simulink model "MATE_SynchronousMachine"  (R2024b)
settings: Solver=FixedStepDiscrete  StartTime=0.0  StopTime=6  FixedStep=Ts  RelTol=1e-4  EnableMultiTasking=on
PostLoadFcn:
  | Ts=25e-6;offset=4;
InitFcn:
  | Ts=25e-6;offset=4;
undefined symbols (not defined in the file): DiscIntNeverNeededParam, MATE, Phase, Rsnu, Single
libraries: fl_lib x79, nesl_utility x53, ee_lib x16, simetran x5, powerlib_extras x3, simulink_extras x2, simulink x2
(part 3 of 5)

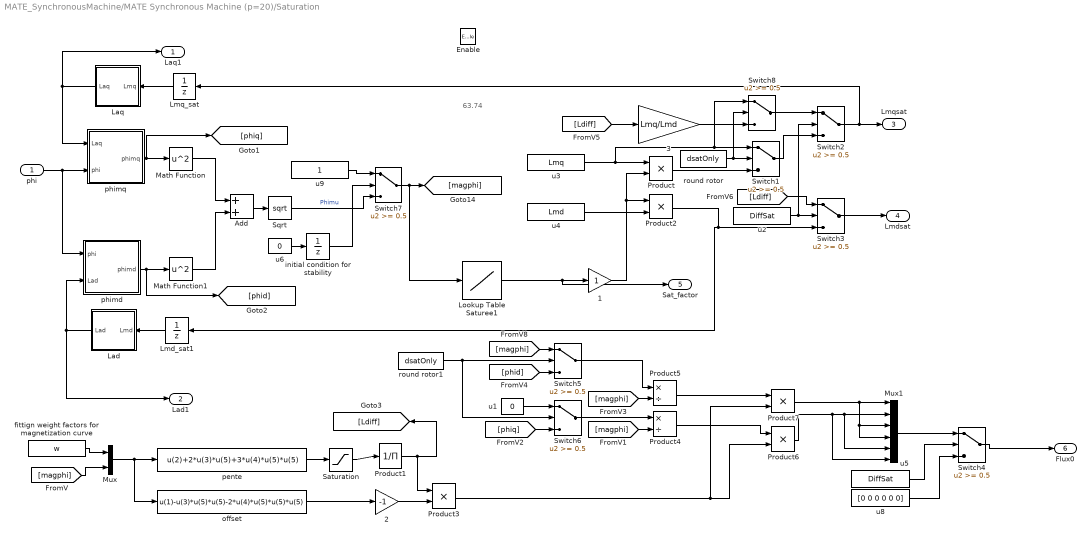
== system MATE_SynchronousMachine/MATE Synchronous Machine (p=20)/Saturation ==
  note: 63.74
  phi : Inport
  Enable : EnablePort
  1 : Gain  SaturateOnIntegerOverflow=on  OutDataTypeStr=Inherit: Same as input  ParamDataTypeStr=Inherit: Same as input
  2 : Gain  Gain=-1  SaturateOnIntegerOverflow=on  OutDataTypeStr=Inherit: Same as input  ParamDataTypeStr=Inherit: Same as input
  3 : Gain  Gain=Lmq/Lmd  SaturateOnIntegerOverflow=on  OutDataTypeStr=Inherit: Same as input  ParamDataTypeStr=Inherit: Same as input
  Add : Sum
  Lad : Subsystem
  Laq : Subsystem
  Lmd_sat1 : UnitDelay  InitialCondition=Lmd  SampleTime=Ts  HasFrameUpgradeWarning=on
  Lmq_sat : UnitDelay  InitialCondition=Lmq  SampleTime=Ts  HasFrameUpgradeWarning=on
  Lookup Table Saturee1 : Lookup  InputValues=table_flux_input  Table=table_saturation_factor  SaturateOnIntegerOverflow=off
  Math Function : Math  Operator=square  SignedPower=on
  Math Function1 : Math  Operator=square  SignedPower=on
  Mux : Mux  Inputs=2
  Mux1 : Mux  Inputs=6
  Product{,2..3,6..7} (5 alike) : Product  RndMeth=Zero
  Product1 : Product  Inputs=/  RndMeth=Zero
  Product4 : Product  Inputs=*/  RndMeth=Zero
  Product5 : Product  Inputs=*/  RndMeth=Zero
  Saturation : Saturate  UpperLimit=inf  LowerLimit=1e-7
  Sqrt : Sqrt  OutputSignalType=real
  Switch{1..8} (8 alike) : Switch  Threshold=0.5  SaturateOnIntegerOverflow=off  InputSameDT=off
  fittign weight factors for magnetization curve : Constant  Value=w
  initial condition for stability : UnitDelay  InitialCondition=1  SampleTime=Ts  HasFrameUpgradeWarning=on
  offset : Fcn  Expr=u(1)-u(3)*u(5)*u(5)-2*u(4)*u(5)*u(5)*u(5)
  pente : Fcn  Expr=u(2)+2*u(3)*u(5)+3*u(4)*u(5)*u(5)
  phimd : Subsystem
  phimq : Subsystem
  round rotor : Constant  Value=dsatOnly
  round rotor1 : Constant  Value=dsatOnly
  u1 : Constant  Value=0
  u2 : Constant  Value=DiffSat
  u3 : Constant  Value=Lmq
  u4 : Constant  Value=Lmd
  u5 : Constant  Value=DiffSat
  u6 : Constant  Value=0
  u8 : Constant  Value=[0 0 0 0 0 0]
  u9 : Constant
  Laq1 : Outport
  Lad1 : Outport  Port=2
  Lmqsat : Outport  Port=3
  Lmdsat : Outport  Port=4
  Sat_factor : Outport  Port=5
  Flux0 : Outport  Port=6
  wires:
  u6/1 -> initial condition for stability/1
  Product2/1 -> Lmd_sat1/1, Switch3/3
  u4/1 -> Product2/2
  u3/1 -> Product/1, Switch1/1, Switch8/1
  Sqrt/1 -> Switch7/3  "Phimu"
  Math Function1/1 -> Add/2
  Math Function/1 -> Add/1
  Add/1 -> Sqrt/1
  phi/1 -> phimd/1(phi), phimq/2(phi)
  Lad/1(Lad) -> Lad1/1, phimd/2(Lad)
  phimd/1(phimd) -> [phid], Math Function1/1
  Lmd_sat1/1 -> Lad/1(Lmd)
  Laq/1(Laq) -> phimq/1(Laq), Laq1/1
  phimq/1(phimq) -> [phiq], Math Function/1
  Lmq_sat/1 -> Laq/1(Lmq)
  round rotor/1 -> Switch1/2, Switch8/2
  Product/1 -> Switch1/3
  Switch1/1 -> Switch2/3
  1/1 -> Product/2, Product2/1
  Lookup Table Saturee1/1 -> 1/1, Sat_factor/1
  fittign weight factors for magnetization curve/1 -> Mux/1
  [magphi] -> Mux/2
  Mux/1 -> pente/1, offset/1
  Product1/1 -> [Ldiff], Product3/1
  offset/1 -> 2/1
  2/1 -> Product3/2
  Product3/1 -> Product7/2, Product6/2
  [magphi] -> Product4/2
  [magphi] -> Product5/2
  Product6/1 -> Mux1/2, Mux1/5, Mux1/6
  Product7/1 -> Mux1/1, Mux1/3, Mux1/4
  Product5/1 -> Product7/1
  Product4/1 -> Product6/1
  Switch3/1 -> Lmdsat/1
  Switch2/1 -> Lmq_sat/1, Lmqsat/1
  u2/1 -> Switch3/2, Switch2/2
  [Ldiff] -> 3/1
  [Ldiff] -> Switch3/1
  Mux1/1 -> Switch4/1
  Switch4/1 -> Flux0/1
  u5/1 -> Switch4/2
  u8/1 -> Switch4/3
  pente/1 -> Saturation/1
  Saturation/1 -> Product1/1
  u9/1 -> Switch7/1
  Switch7/1 -> [magphi], Lookup Table Saturee1/1
  initial condition for stability/1 -> Switch7/2
  [phid] -> Switch5/3
  [phiq] -> Switch6/3
  Switch5/1 -> Product5/1
  Switch6/1 -> Product4/1
  [magphi] -> Switch5/1
  u1/1 -> Switch6/1
  round rotor1/1 -> Switch6/2, Switch5/2
  Switch8/1 -> Switch2/1
  3/1 -> Switch8/3

== system MATE_SynchronousMachine/MATE Synchronous Machine (p=20)/Update Matrix L (with Lcanay) ==
  Lmq : Inport
  Lmd : Inport  Port=2
  Ll : Inport  Port=3
  Selector1 : Selector  NumberOfDimensions=2  InputPortWidth=3  IndexOptions=Index vector (dialog),Index vector (dialog)  Indices=[1:nb_row],[1:nb_row]  OutputSizes=1,1
  Selector8 : Selector  NumberOfDimensions=2  InputPortWidth=3  IndexOptions=Index vector (dialog),Index vector (dialog)  Indices=[1:nb_row],[1:nb_row]  OutputSizes=1,1
  Sum1 : Sum  SaturateOnIntegerOverflow=on
  Sum2 : Sum  SaturateOnIntegerOverflow=on
  Update Lmd rows[1] col[1] : Assignment  NumberOfDimensions=2  IndexOptions=Index vector (dialog),Index vector (dialog)  Indices=[1 3 4],[1 3 4]  OutputSizes=1,1
  "Update Lmq rows[1,5, (6)] col[1,5, (6)] " : Assignment  NumberOfDimensions=2  IndexOptions=Index vector (dialog),Index vector (dialog)  Indices=[2 5 6],[2 5 6]  OutputSizes=1,1
  u1 : Constant  Value="[0 0 0 0 0 0; 0 0 0 0 0 0; 0 0 Lcanay Lcanay 0 0; 0 0 Lcanay Lcanay 0 0; 0 0 0 0 0 0; 0 0  0 0 0 0]"
  u3 : Constant  Value=zeros(6,6)
  Lsat : Outport
  wires:
  Sum1/1 -> Sum2/1
  Update Lmd rows[1] col[1]/1 -> Sum1/1
  Selector1/1 -> Sum1/2
  u1/1 -> Selector1/1
  "Update Lmq rows[1,5, (6)] col[1,5, (6)] "/1 -> Selector8/1
  Lmq/1 -> "Update Lmq rows[1,5, (6)] col[1,5, (6)] "/2
  u3/1 -> "Update Lmq rows[1,5, (6)] col[1,5, (6)] "/1
  Lmd/1 -> Update Lmd rows[1] col[1]/2
  Ll/1 -> Sum2/2
  Sum2/1 -> Lsat/1
  Selector8/1 -> Update Lmd rows[1] col[1]/1

== system MATE_SynchronousMachine/MATE Synchronous Machine (p=20)/inverse ==
  Lsat : Inport
  Enable : EnablePort
  Gain8 : Gain  Gain=-1
  Goto1 : Goto  Commented=on  GotoTag=invL
  Product3 : Product  Multiplication=Matrix(*)  SaturateOnIntegerOverflow=on  OutDataTypeStr=Inherit: Same as first input
  Rwinding : Constant  Value="[Rs 0 0 0 0 0; 0 Rs 0 0 0 0; 0 0 Rf  0 0 0; 0 0 0 Rkd 0 0; 0 0 0 0  Rkq 0; 0 0 0 0 0 Rkq2]"
  Selector8 : Selector  NumberOfDimensions=2  InputPortWidth=3  IndexOptions=Index vector (dialog),Index vector (dialog)  Indices=[1:nb_row],[1:nb_row]  OutputSizes=1,1
  inversion2 : Product  Inputs=/  Multiplication=Matrix(*)  RndMeth=Zero
  -R*inv(L) : Outport
  inv(L) : Outport  Port=2
  wires:
  Gain8/1 -> Product3/1
  inversion2/1 -> Goto1/1, Product3/2, inv(L)/1
  Lsat/1 -> inversion2/1
  Selector8/1 -> Gain8/1
  Rwinding/1 -> Selector8/1
  Product3/1 -> -R*inv(L)/1

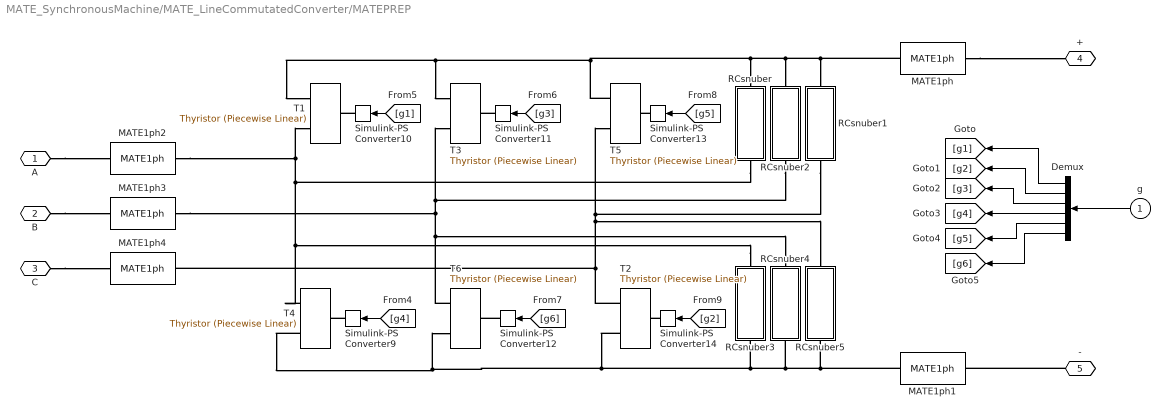
== system MATE_SynchronousMachine/MATE_LineCommutatedConverter/MATEPREP ==
  g : Inport
  Demux : Demux  Outputs=6
  MATE1ph : simetran/MATE1ph  bn=4  conty=Single-Phase  it=auto  Rse=1e-4  Rsh=1e9
      settings: AttributesFormatString=# %<bn>
  MATE1ph1 : simetran/MATE1ph  bn=5  conty=Single-Phase  it=auto  Rse=1e-4  Rsh=1e9
      settings: AttributesFormatString=# %<bn>
  MATE1ph2 : simetran/MATE1ph  bn=1  conty=Single-Phase  it=auto  Rse=1e-4  Rsh=1e9
      settings: AttributesFormatString=# %<bn>
  MATE1ph3 : simetran/MATE1ph  bn=2  conty=Single-Phase  it=auto  Rse=1e-4  Rsh=1e9
      settings: AttributesFormatString=# %<bn>
  MATE1ph4 : simetran/MATE1ph  bn=3  conty=Single-Phase  it=auto  Rse=1e-4  Rsh=1e9
      settings: AttributesFormatString=# %<bn>
  RCsnuber : Subsystem
  RCsnuber1 : Subsystem
  RCsnuber2 : Subsystem
  RCsnuber3 : Subsystem
  RCsnuber4 : Subsystem
  RCsnuber5 : Subsystem
  Simulink-PS Converter{9..14} (6 alike) : nesl_utility/Simulink-PS Converter  PhysicalDomain=network_engine_domain  SubClassName=ps_input  LeftPortType=input  RightPortType=output  PseudoPeriodic=off  Frequencies=[]  NoiseDistribution=none  NoiseParameters=[]  Unit=1  AffineConversion=off  FilteringAndDerivatives=provide  SimscapeFilterOrder=1  InputFilterTimeConstant=0.001  UdotUserProvided=0
  T{1..6} (6 alike) : ee_lib/Semiconductors & Converters/Thyristor (Piecewise Linear)  port_option=ee.enum.controlport.ps  Vf=0.8 V  Ron=0.001 Ohm  Goff=1e-5 1/Ohm  Vgt=0.5 V  Ih=1 A  diode_param=ee.enum.semiconductors.protectionDiode.external  diode_Vf=0.8 V  diode_Ron=0.001 Ohm  diode_Goff=1e-5 1/Ohm  diode_C=50e-9 F  diode_iRM=-235 A  diode_iF=300 A  diode_idot=-50 A/us  diode_trr_param=ee.enum.converters.diodetrr.trr_factor  diode_trr_factor=3  diode_trr=15 us  diode_Qrr=1500 s*uA  iak_specify=off  iak_priority=None  iak=0 A  iak_nominal_specify=off  iak_nominal_value=1  iak_nominal_unit=A  vak_specify=off  vak_priority=None  vak=0 V  vak_nominal_specify=off  vak_nominal_value=1  vak_nominal_unit=V  vgk_specify=off  vgk_priority=None  vgk=0 V  vgk_nominal_specify=off  vgk_nominal_value=1  vgk_nominal_unit=V  thermal_loss_option=ee.enum.converters.thermalLossOption.constantvalues  Von_data=[0, .1, .6, .8, 1, 1.3, 1.6, 2, 2.4; 0, .1, .7, 1, 1.2, 1.5, 1.9, 2.4, 2.8] V  Tj=[298.15, 398.15] K  Iout_data=[0, .1, 1, 5, 10, 20, 40, 70, 100] A  Eon_data=[0, .0024, .024, .12, .2, .48, 1.04, 2.16, 3.24; 0, .003, .03, .15, .25, .6, 1.3, 2.7, 4.05] * 1e-3 J  Tj_loss=[298.15, 398.15] K  Iout_data_loss=[0, .1, 1, 5, 10, 20, 40, 70, 100] A  Eon_scalar=22.86e-3 J  Eoff_natural_commutation=10e-3 J  Voff=300 V  Iout_scalar=600 A  onCurrentMeasDelay=1e-4 s  diodeModelType=ee.enum.converters.diodeModelType.pwl  diodeTableType=ee.enum.diode.tableType.IfMat  diode_IfMat=[.07, .12, .19, 1.75, 4.24, 7.32, 11.2; .16, .3, .72, 2.14, 4.02, 6.35, 9.12] A  diode_VfMat=[.9, 1.15, 1.25, 1.5, 1.75, 2.17, 2.6, 2.85; .58, .68, .75, 1.1, 1.38, 1.77, 2.27, 2.7] V  diode_TjVec=[25, 125] degC  diode_VfVec=[.5, .7, .9, 1.3, 1.7, 2.1, 2.5] V  diode_IfVec=[.1, .2, .5, 1, 2, 4, 7, 10] A  diode_rec_loss_model=ee.enum.diode.reverseRecoveryModel.fixed  diode_ErecVal=0 J  diode_scaleWithIandV=true  diode_ErecMat=zeros(2, 3) J  diode_TjrecVec=[298.15, 398.15] K  diode_IfrecVec=[.1, 1, 10] A  diode_IrecVal=10 A  diode_VrecVal=10 V  diode_tFilter=1 / 1000 / 100 s  thermal_network_parameterization=ee.enum.thermalNetworkTopology.external  Rth=[.08, .5] K/W  Rth_Cauer=[.08, .1, .5] K/W  Rth_Foster=[.08, .14, .22, .16] K/W  thermal_mass_parameterization=ee.enum.thermalNetwork.timeconstant  thermal_mass=[.01, .5] J/K  thermal_mass_Cauer=[.01, .1, .5] J/K  thermal_mass_Foster=[.001, .005, .05, .5] J/K  thermal_time_constant=[.001, .2] s  thermal_time_constant_Cauer=[.001, .1, .2] s  thermal_time_constant_Foster=[7e-05, .0007, .01, .08] s  thermal_mass_initial_temperatures=[25, 25] degC  thermal_mass_initial_temperatures_Cauer=[25, 25, 25] degC  junction_thermal_mass=0.01 J/K  Tvec_initial_Foster=[25, 25, 25, 25] degC  junction_temperature_specify=off  junction_temperature_priority=None  junction_temperature=25 degC  junction_temperature_nominal_specify=off  junction_temperature_nominal_value=1  junction_temperature_nominal_unit=degC  Qj_specify=off  Qj_priority=None  Qj=0 W  Qj_nominal_specify=off  Qj_nominal_value=1  Qj_nominal_unit=W  accumulatedSwitchingLosses_specify=off  accumulatedSwitchingLosses_priority=None  accumulatedSwitchingLosses=0 J
      settings: InternalSimscapePortConfiguration="{\"Bottom\":[],\"Left\":[{\"id\":\"G\",\"label\":\"\",\"type\":\"input\"}],\"Right\":[{\"id\":\"A\",\"label\":\"\",\"type\":\"foundation.electrical.electrical\"},{\"id\":\"K\",\"label\":\"\",\"type\":\"foundation.electrical.electrical\"}],\"Top\":[]}"
  A : PMIOPort  Side=Left
  B : PMIOPort  Port=2  Side=Left
  C : PMIOPort  Port=3  Side=Left
  + : PMIOPort  Port=4  Side=Right
  - : PMIOPort  Port=5  Side=Right
  wires:
  Demux/5 -> [g5]
  Demux/6 -> [g6]
  Demux/4 -> [g4]
  Demux/3 -> [g3]
  Demux/2 -> [g2]
  Demux/1 -> [g1]
  g/1 -> Demux/1
  [g4] -> Simulink-PS Converter9/1
  [g1] -> Simulink-PS Converter10/1
  [g3] -> Simulink-PS Converter11/1
  [g6] -> Simulink-PS Converter12/1
  [g5] -> Simulink-PS Converter13/1
  [g2] -> Simulink-PS Converter14/1
  connections:
  RCsnuber3/LConn1 -- T4/RConn2 -- RCsnuber/RConn1 -- MATE1ph2/RConn1 -- T1/RConn1
  MATE1ph3/RConn1 -- RCsnuber2/RConn1 -- T3/RConn1 -- T6/RConn2 -- RCsnuber4/LConn1
  RCsnuber1/RConn1 -- T5/RConn1 -- T2/RConn2 -- MATE1ph4/RConn1 -- RCsnuber5/LConn1
  RCsnuber4/RConn1 -- MATE1ph1/RConn1 -- RCsnuber5/RConn1 -- T2/RConn1 -- T6/RConn1 -- T4/RConn1 -- RCsnuber3/RConn1
  MATE1ph/RConn1 -- T1/RConn2 -- T3/RConn2 -- T5/RConn2 -- RCsnuber/LConn1 -- RCsnuber2/LConn1 -- RCsnuber1/LConn1
  -/RConn1 -- MATE1ph1/LConn1
  A/RConn1 -- MATE1ph2/LConn1
  B/RConn1 -- MATE1ph3/LConn1
  C/RConn1 -- MATE1ph4/LConn1
  Simulink-PS Converter9/RConn1 -- T4/LConn1
  Simulink-PS Converter10/RConn1 -- T1/LConn1
  Simulink-PS Converter11/RConn1 -- T3/LConn1
  Simulink-PS Converter12/RConn1 -- T6/LConn1
  Simulink-PS Converter13/RConn1 -- T5/LConn1
  Simulink-PS Converter14/RConn1 -- T2/LConn1
  MATE1ph/LConn1 -- +/RConn1

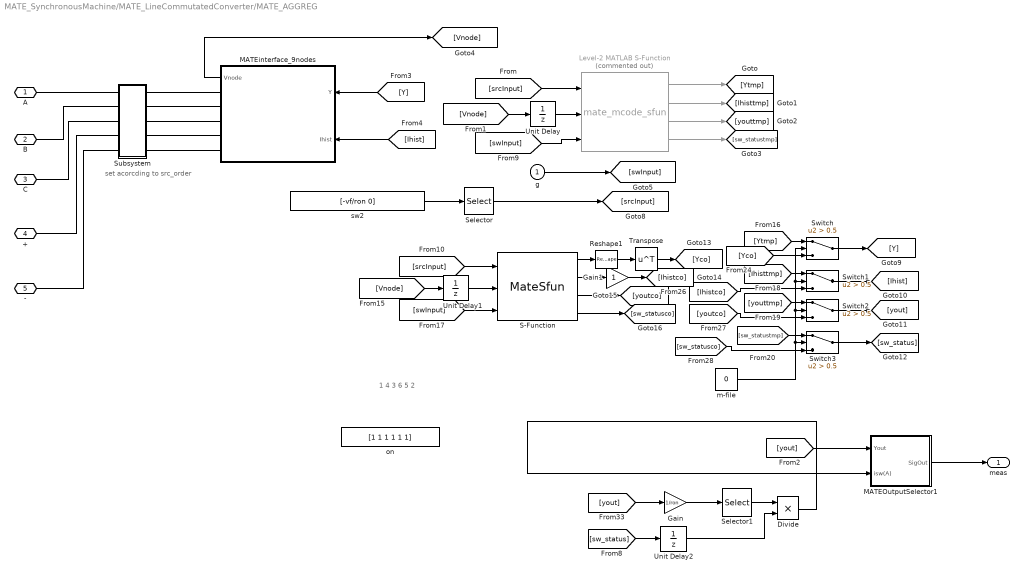
== system MATE_SynchronousMachine/MATE_LineCommutatedConverter/MATE_AGGREG ==
  note: set acorcding to src_order
  note: 1 4 3 6 5 2
  g : Inport
  Divide : Product
  Gain : Gain  Gain=1/ron
  Gain1 : Gain
  Level-2 MATLAB S-Function : M-S-Function  Commented=on  FunctionName=mate_mcode_sfun  Parameters=MATE,vf
  MATEOutputSelector1 : Subsystem
  MATEinterface_9nodes : Subsystem
  Reshape1 : Reshape  OutputDimensionality=Customize  OutputDimensions=[MATE.NumberOfNodes,MATE.NumberOfNodes]
  S-Function : S-Function  FunctionName=MateSfun  Parameters="MATERT.sizes,MATERT.As  ,MATERT.Bs,MATERT.Cs,MATERT.Ds,MATERT.Rsw,MATERT.SwType,MATERT.DISC,MATERT.h,MATERT.U0,MATERT.X0,vf"  SFunctionDeploymentMode=off  EnableBusSupport=off
  Selector : Selector  InputPortWidth=2  IndexOptions=Index vector (dialog)  Indices="[1 1 1 1 1 1  2 2 2 2 2]"  OutputSizes=1
  Selector1 : Selector  InputPortWidth=11  IndexOptions=Index vector (dialog)  Indices=[1 2 3 4 5 6]  OutputSizes=1
  Subsystem : Subsystem
  Switch{,1..3} (4 alike) : Switch  Criteria=u2 > Threshold  Threshold=0.5  SaturateOnIntegerOverflow=off  InputSameDT=off
  Transpose : Math  Operator=transpose
  Unit Delay : UnitDelay  SampleTime=Ts  HasFrameUpgradeWarning=on
  Unit Delay1 : UnitDelay  SampleTime=Ts  HasFrameUpgradeWarning=on
  Unit Delay2 : UnitDelay  SampleTime=Ts  HasFrameUpgradeWarning=on
  m-file : Constant  Value=0
  on : Constant  Value=[1 1 1 1 1 1]
  sw2 : Constant  Value=[-vf/ron 0]
  A : PMIOPort  Side=Left
  B : PMIOPort  Port=2  Side=Left
  C : PMIOPort  Port=3  Side=Left
  + : PMIOPort  Port=4  Side=Right
  - : PMIOPort  Port=5  Side=Right
  meas : Outport
  wires:
  m-file/1 -> Switch3/2, Switch/2, Switch1/2, Switch2/2
  Level-2 MATLAB S-Function/1 -> [Ytmp]
  Unit Delay/1 -> Level-2 MATLAB S-Function/2
  [swInput] -> S-Function/3
  S-Function/3 -> [youtco]
  Level-2 MATLAB S-Function/2 -> [Ihisttmp]
  Level-2 MATLAB S-Function/3 -> [youttmp]
  [youtco] -> Switch2/3
  [sw_statustmp] -> Switch3/1
  [Vnode] -> Unit Delay1/1
  [youttmp] -> Switch2/1
  [srcInput] -> Level-2 MATLAB S-Function/1
  Gain1/1 -> [Ihistco]
  [Ihistco] -> Switch1/3
  [Ytmp] -> Switch/1
  [Ihist] -> MATEinterface_9nodes/2(Ihist)
  [Vnode] -> Unit Delay/1
  [srcInput] -> S-Function/1
  Unit Delay1/1 -> S-Function/2
  S-Function/1 -> Reshape1/1
  S-Function/2 -> Gain1/1
  Switch2/1 -> [yout]
  Transpose/1 -> [Yco]
  Reshape1/1 -> Transpose/1
  S-Function/4 -> [sw_statusco]
  Switch/1 -> [Y]
  [Ihisttmp] -> Switch1/1
  [sw_statusco] -> Switch3/3
  MATEinterface_9nodes/1(Vnode) -> [Vnode]
  [swInput] -> Level-2 MATLAB S-Function/3
  [Yco] -> Switch/3
  Switch1/1 -> [Ihist]
  [Y] -> MATEinterface_9nodes/1(Y)
  Switch3/1 -> [sw_status]
  Level-2 MATLAB S-Function/4 -> [sw_statustmp]
  sw2/1 -> Selector/1
  Selector/1 -> [srcInput]
  Divide/1 -> MATEOutputSelector1/2(isw(A))
  Selector1/1 -> Divide/1
  [sw_status] -> Unit Delay2/1
  [yout] -> MATEOutputSelector1/1(Yout)
  Gain/1 -> Selector1/1
  Unit Delay2/1 -> Divide/2
  [yout] -> Gain/1
  MATEOutputSelector1/1(SigOut) -> meas/1
  g/1 -> [swInput]
  connections:
  Subsystem/RConn1 -- MATEinterface_9nodes/RConn1
  B/RConn1 -- Subsystem/LConn2
  A/RConn1 -- Subsystem/LConn1
  C/RConn1 -- Subsystem/LConn3
  +/RConn1 -- Subsystem/LConn4
  -/RConn1 -- Subsystem/LConn5
  Subsystem/RConn2 -- MATEinterface_9nodes/RConn2
  Subsystem/RConn3 -- MATEinterface_9nodes/RConn3
  Subsystem/RConn4 -- MATEinterface_9nodes/RConn4
  Subsystem/RConn5 -- MATEinterface_9nodes/RConn5

== system MATE_SynchronousMachine/Mesure et visualisation/Discrete Mean value ==
  In : Inport
  Constant : Constant  Value=Vinit  SampleTime=Ts
  Discrete Variable Transport Delay : powerlib_extras/Discrete  Control Blocks/Discrete Variable Transport Delay  MaxDelay=Delay+Ts  InitialValue=0  Ts=Ts
  Gain : Gain  Gain=K1  SaturateOnIntegerOverflow=on  OutDataTypeStr=Inherit: Same as input  ParamDataTypeStr=Inherit: Same as input
  Gain1 : Gain  Gain=K2  SaturateOnIntegerOverflow=on  OutDataTypeStr=Inherit: Same as input  ParamDataTypeStr=Inherit: Same as input
  Integ4 : DiscreteIntegrator  IntegratorMethod=Integration: Trapezoidal  SampleTime=Ts  ICPrevOutput=DiscIntNeverNeededParam  ICPrevScaledInput=DiscIntNeverNeededParam
  K1 : Constant  Value=Delay  SampleTime=Ts
  K2 : Constant  Value=Freq  SampleTime=Ts
  Product : Product  InputSameDT=on  SaturateOnIntegerOverflow=on  OutDataTypeStr=Inherit: Same as first input
  Step : Step  Time=1/Freq  SampleTime=Ts
  Sum1 : Sum  Inputs=+-  InputSameDT=on  SaturateOnIntegerOverflow=on  OutDataTypeStr=Inherit: Same as first input
  Sum5 : Sum  InputSameDT=on  SaturateOnIntegerOverflow=on  OutDataTypeStr=Inherit: Same as first input
  Sum7 : Sum  Inputs=-+  InputSameDT=on  SaturateOnIntegerOverflow=on  OutDataTypeStr=Inherit: Same as first input
  Switch : Switch  Threshold=0.5  SaturateOnIntegerOverflow=off
  Unit Delay : UnitDelay  SampleTime=Ts  HasFrameUpgradeWarning=on
  Mean : Outport  VectorParamsAs1DForOutWhenUnconnected=off
  wires:
  Product/1 -> Sum5/1  "Mean value"
  Sum7/1 -> Product/1
  Integ4/1 -> Discrete Variable Transport Delay/1, Sum7/2
  K2/1 -> Product/2
  In/1 -> Integ4/1, Gain1/1, Unit Delay/1  "In"
  Sum5/1 -> Switch/1
  Step/1 -> Switch/2
  Constant/1 -> Switch/3
  Switch/1 -> Mean/1
  Discrete Variable Transport Delay/1 -> Sum7/1
  K1/1 -> Discrete Variable Transport Delay/2
  Gain1/1 -> Sum1/1
  Unit Delay/1 -> Gain/1
  Gain/1 -> Sum1/2
  Sum1/1 -> Sum5/2  "Correction"

== system MATE_SynchronousMachine/turbine1/Hydraulic Turbine and Governor ==
  wref : Inport
  Pref : Inport  Port=2
  we : Inport  Port=3
  Pe0 : Inport  Port=4
  dw : Inport  Port=5
  Model : Subsystem  mask(Discrete Hydraulic Turbine and Governor){sm=sm, gate=gate, reg=reg, hyd=hyd, dref=dref, po=po, Ts=Ts}
      mask prompts: sm "Servo-motor [ Ka()  Ta(sec) ]:"; gate "Gate opening limits [ gmin,gmax(pu)    vgmin,vgmax(pu/s) ]:"; reg "Permanent droop and regulator  [ Rp() Kp() Ki() Kd() Td(s) ]:"; hyd "Hydraulic turbine [ beta()  Tw(sec) ]:"; dref "Droop reference (0=power error, 1=gate opening):"; po "Initial mechanical power (pu):"; Ts "Sample time:"
      mask help:
      | Implements a discrete hydraulic turbine combined to a discrete PID governor system.
      |
      | 1st input: desired speed (p.u.);
      | 2nd input: desired electrical power (p.u.);
      | 3rd input: synchronous machine's actual speed (p.u., measurement output 13 of SM block);
      | 4th input: synchronous machine's actual electrical power (p.u., measurement output 14 of SM block);
      | 5th input: synchronous machine's actual speed deviation with respect to nominal (%, measurement output 15 of SM block);
      |
      | 1st output: mechanical power to be applied to the Synchronous Machine block's 1st input (p.u.);
      | 2nd output: gate opening (p.u.).
      mask init:
      | ka=sm(1);ta=sm(2);gmin=gate(1);gmax=gate(2);vgmin=gate(3);vgmax=gate(4);Rp=reg(1);kp=reg(2);ki=reg(3);kd=reg(4);td=reg(5);beta=hyd(1);tw=hyd(2);go=po*(gmax-gmin);
      mask Help: helpview(psbhelp);
  Pm : Outport  InitialOutput=0  VectorParamsAs1DForOutWhenUnconnected=off
  gate : Outport  Port=2  InitialOutput=0  VectorParamsAs1DForOutWhenUnconnected=off
  wires:
  wref/1 -> Model/1(wref)
  Pref/1 -> Model/2(Pref)
  we/1 -> Model/3(we)
  Pe0/1 -> Model/4(Pe)
  dw/1 -> Model/5(dw)
  Model/2(gate) -> gate/1
  Model/1(Pm) -> Pm/1

== system MATE_SynchronousMachine/turbine1/Mechanical model ==
  Te : Inport  PortDimensions=1
  Pin : Inport  Port=2
  1 ----- J : Gain  Gain=1/J  SaturateOnIntegerOverflow=on  OutDataTypeStr=Inherit: Same as input  ParamDataTypeStr=Inherit: Same as input
  Delay Prediction : Subsystem
  Divide : Product  Inputs=/*
  F : Gain  Gain=F  SaturateOnIntegerOverflow=on  OutDataTypeStr=Inherit: Same as input  ParamDataTypeStr=Inherit: Same as input
  Rotor speed deviation (dw) : DiscreteIntegrator  InitialCondition=fo*2*pi  SampleTime=Ts  ICPrevOutput=DiscIntNeverNeededParam  ICPrevScaledInput=DiscIntNeverNeededParam
  Sum2 : Sum  Inputs=+--  InputSameDT=on  SaturateOnIntegerOverflow=on  OutDataTypeStr=Inherit: Same as first input
  wmec : Outport  InitialOutput=0
  delta_wm : Outport  Port=2  InitialOutput=0
  wires:
  Rotor speed deviation (dw)/1 -> delta_wm/1, F/1, Divide/1, wmec/1, Delay Prediction/1(in)  "dw"
  1 ----- J/1 -> Rotor speed deviation (dw)/1
  Divide/1 -> Sum2/1
  Te/1 -> Sum2/2  "Te"
  F/1 -> Sum2/3
  Sum2/1 -> 1 ----- J/1
  Pin/1 -> Divide/2  "Pm"

== system MATE_SynchronousMachine/Command/Regulateur de courant/Discrete 1st-Order Filter ==
  In : Inport
  Discrete State-Space : DiscreteStateSpace  A=Ad  B=Bd  C=Cd  D=Dd  InitialCondition=x0d  SampleTime=Ts
  Out : Outport  InitialOutput=0  VectorParamsAs1DForOutWhenUnconnected=off
  wires:
  In/1 -> Discrete State-Space/1
  Discrete State-Space/1 -> Out/1

== system MATE_SynchronousMachine/Command/Regulateur de courant/Discrete PI Controller1 ==
  Error : Inport  SampleTime=Ts
  Discrete-Time Integrator : DiscreteIntegrator  InitialCondition=Init  SampleTime=Ts  LimitOutput=on  UpperSaturationLimit=UpperLimit  LowerSaturationLimit=LowerLimit  ICPrevOutput=DiscIntNeverNeededParam  ICPrevScaledInput=DiscIntNeverNeededParam
  Kp4 : Gain  Gain=Kp  SaturateOnIntegerOverflow=on  SampleTime=Ts  OutDataTypeStr=Inherit: Same as input  ParamDataTypeStr=Inherit: Same as input
  Kp5 : Gain  Gain=Ki  SaturateOnIntegerOverflow=on  SampleTime=Ts  OutDataTypeStr=Inherit: Same as input  ParamDataTypeStr=Inherit: Same as input
  Saturation2 : Saturate  UpperLimit=UpperLimit  LowerLimit=LowerLimit  SampleTime=Ts
  Sum6 : Sum  InputSameDT=on  SaturateOnIntegerOverflow=on  SampleTime=Ts  OutDataTypeStr=Inherit: Same as first input
  Zero-Order Hold : ZeroOrderHold  SampleTime=Ts
  Out : Outport  SampleTime=Ts  InitialOutput=0  VectorParamsAs1DForOutWhenUnconnected=off
  wires:
  Zero-Order Hold/1 -> Sum6/1
  Saturation2/1 -> Out/1
  Discrete-Time Integrator/1 -> Sum6/2
  Kp4/1 -> Zero-Order Hold/1
  Kp5/1 -> Discrete-Time Integrator/1
  Sum6/1 -> Saturation2/1
  Error/1 -> Kp5/1, Kp4/1

== system MATE_SynchronousMachine/Command/Regulateur de tension (Mode automatique)/Discrete PI Controller1 ==
  Error : Inport  SampleTime=Ts
  Discrete-Time Integrator : DiscreteIntegrator  InitialCondition=Init  SampleTime=Ts  LimitOutput=on  UpperSaturationLimit=UpperLimit  LowerSaturationLimit=LowerLimit  ICPrevOutput=DiscIntNeverNeededParam  ICPrevScaledInput=DiscIntNeverNeededParam
  Kp4 : Gain  Gain=Kp  SaturateOnIntegerOverflow=on  SampleTime=Ts  OutDataTypeStr=Inherit: Same as input  ParamDataTypeStr=Inherit: Same as input
  Kp5 : Gain  Gain=Ki  SaturateOnIntegerOverflow=on  SampleTime=Ts  OutDataTypeStr=Inherit: Same as input  ParamDataTypeStr=Inherit: Same as input
  Saturation2 : Saturate  UpperLimit=UpperLimit  LowerLimit=LowerLimit  SampleTime=Ts
  Sum6 : Sum  InputSameDT=on  SaturateOnIntegerOverflow=on  SampleTime=Ts  OutDataTypeStr=Inherit: Same as first input
  Zero-Order Hold : ZeroOrderHold  SampleTime=Ts
  Out : Outport  SampleTime=Ts  InitialOutput=0  VectorParamsAs1DForOutWhenUnconnected=off
  wires:
  Zero-Order Hold/1 -> Sum6/1
  Saturation2/1 -> Out/1
  Discrete-Time Integrator/1 -> Sum6/2
  Kp4/1 -> Zero-Order Hold/1
  Kp5/1 -> Discrete-Time Integrator/1
  Sum6/1 -> Saturation2/1
  Error/1 -> Kp5/1, Kp4/1

== system MATE_SynchronousMachine/Command/Regulateur de tension (Mode automatique)/Discrete 3-phase Positive-Sequence Fundamental Value ==
  note: Discrete Measurement - Positive-sequence Fundamental Value
  abc : Inport  PortDimensions=3
  Cartesian to Polar : simulink_extras/Transformations/Cartesian to Polar
  Demux : Demux  Outputs=3
      settings: DisplayOption=none
  Discrete Mean value1 : Subsystem  mask(Discrete Mean value){Freq=Freq, Vinit=Real_Init, Ts=Ts}
      mask prompts: Freq "Fundamental frequency (Hz):"; Vinit "Initial input (DC component):"; Ts "Sample time:"
      mask help: Compute the mean value of the input signal over a running window of one cycle of the specified fundamental frequency.
      mask init: same as MATE_SynchronousMachine/Mesure et visualisation/Discrete Mean value
      mask Display: disp('Mean\n(discrete)')
  Discrete Mean value3 : Subsystem  mask(Discrete Mean value){Freq=Freq, Vinit=Imag_Init, Ts=Ts}
      mask prompts: Freq "Fundamental frequency (Hz):"; Vinit "Initial input (DC component):"; Ts "Sample time:"
      mask help: Compute the mean value of the input signal over a running window of one cycle of the specified fundamental frequency.
      mask init: same as MATE_SynchronousMachine/Mesure et visualisation/Discrete Mean value
      mask Display: disp('Mean\n(discrete)')
  Gain : Gain  Gain=2*pi*Freq  SaturateOnIntegerOverflow=on  OutDataTypeStr=Inherit: Same as input  ParamDataTypeStr=Inherit: Same as input
  Mux : Mux  Inputs=2
  Rad->Deg. : Gain  Gain=180/pi  SaturateOnIntegerOverflow=on  OutDataTypeStr=Inherit: Same as input  ParamDataTypeStr=Inherit: Same as input
  Terminator : Terminator
  Trigonometric Function : Trigonometry
  Trigonometric Function1 : Trigonometry  Operator=cos
  abc_to_dq0 Transformation : Subsystem  mask(abc to dq0 Transformation){}
      mask help: Perform a Park transformation from the three-phase (abc) reference frame to the dq0 reference frame.
      mask init:
      | power_initmask();
      mask Help: helpview(psbhelp);
      mask Display: disp('')
  t : DigitalClock  SampleTime=Ts
  Mag : Outport  VectorParamsAs1DForOutWhenUnconnected=off
  Phase : Outport  Port=2  VectorParamsAs1DForOutWhenUnconnected=off
  wires:
  Cartesian to Polar/2 -> Rad->Deg./1
  Cartesian to Polar/1 -> Mag/1
  Gain/1 -> Trigonometric Function1/1, Trigonometric Function/1
  t/1 -> Gain/1
  abc/1 -> abc_to_dq0 Transformation/1(abc)
  Mux/1 -> abc_to_dq0 Transformation/2(sin_cos)
  Discrete Mean value1/1(Mean) -> Cartesian to Polar/1  "Real"
  Rad->Deg./1 -> Phase/1
  Discrete Mean value3/1(Mean) -> Cartesian to Polar/2  "Real"
  abc_to_dq0 Transformation/1(dq0) -> Demux/1
  Demux/3 -> Terminator/1
  Demux/2 -> Discrete Mean value3/1(In)
  Demux/1 -> Discrete Mean value1/1(In)
  Trigonometric Function/1 -> Mux/1
  Trigonometric Function1/1 -> Mux/2

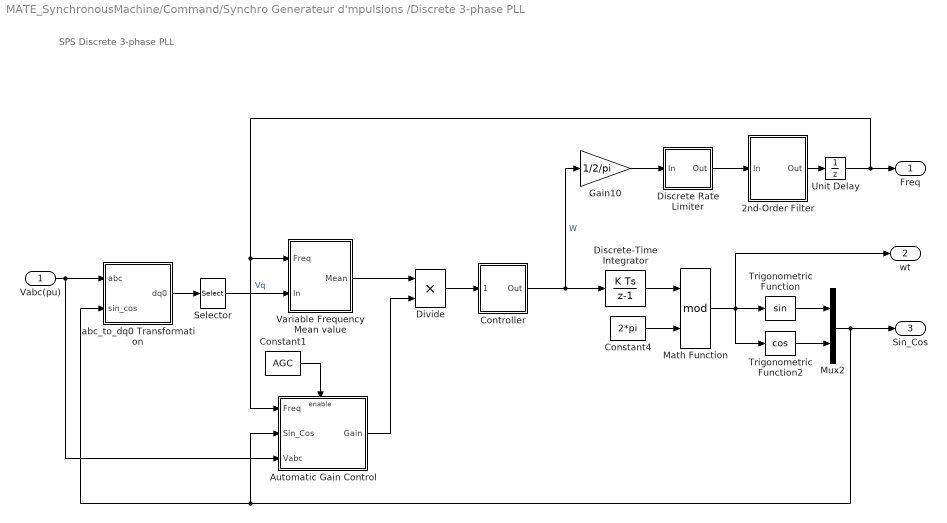
== system MATE_SynchronousMachine/Command/Synchro Generateur d'mpulsions /Discrete 3-phase PLL ==
  note: SPS Discrete 3-phase PLL
  Vabc(pu) : Inport  PortDimensions=3
  2nd-Order Filter : Subsystem  mask(Discrete 2nd-Order Filter){FilterType=Lowpass, Fo=25, Zeta=0.707, Ts=Ts, Initialize=on, Vac_Init=[0 0 Finit], Vdc_Init=Finit, PlotResponse=off, param1=[1 500 0.1]}
      mask prompts: FilterType "Filter Type:"; Fo "Cut-off frequency (Hz):"; Zeta "Damping factor Zeta ( Q = 1 / (2*Zeta) ):"; Ts "Sample time:"; Initialize "Initialize filter states"; Vac_Init "AC initial input: [ Mag  Phase(degrees)  Freq(Hz) ]"; Vdc_Init "DC Initial input:"; PlotResponse "Plot filter response"; param1 "Frequency range(Hz) : [Start  End  Inc.]"
      mask init:
      | str=sprintf(' Fo=%iHz\n\n',Fo);
      | Wo=2*pi*Fo;
      | switch FilterType
      | case 1, % Lowpass
      |        X=[0 1 2 3 4];
      |        Y=[-2 -2 -3 -4 -4];
      |        n2=0;n1=0;n0=Wo*Wo;
      |        d2=1;d1=2*Zeta*Wo;d0=Wo*Wo;
      | 	   Ystep=1;
      |  case 2,   % Highpass
      |        X=[0 1 2 3 4];
      |        Y=[-4 -4 -3 -2 -2];
      |        n2=1;n1=0;n0=0;
      |        d2=1;d1=2*Zeta*Wo;d0=Wo*Wo;
      | 	   Ystep=2;
      |     case 3,   % Bandpass
      |        X=[0 1 2 3 4 5 ];
      |        Y=[-3 -3 -2 -2 -3 -3];
      |        n2=0;n1=2*Zeta*Wo;n0=0;
      |        d2=1;d1=2*Zeta*Wo;d0=Wo*Wo;
      | 	   Ystep=3;
      |     case 4,  %Bandstop (Notch)
      |        X=[0 1 2 3 4 5 ];
      |        Y=[-2 -2 -3 -3 -2 -2];
      |        n2=1;n1=0;n0=Wo*Wo;
      |        d2=1;d1=2*Zeta*Wo;d0=Wo*Wo;
      | 	   Ystep=4;
      |     end
      | %
      | numc=[n2 n1 n0];
      | denc=[d2 d1 d0];
      | [Ac,Bc,Cc,Dc]=tf2ss(numc,denc);
      | %
      | %  Conversion to discrete transfer function
      | nstates = size(Ac,1);
      | invexp = inv(eye(nstates) - (Ts/2)*Ac);
      | Ad = invexp*(eye(nstates) + (Ts/2)*Ac);
      | Bd = invexp*Bc;
      | Cd = Cc*invexp*Ts;
      | Dd = Cc*invexp*Bc*(Ts/2) + Dc;
      | %
      | if Initialize==1  % Compute initial conditions on states
      | u1=Vac_Init(1)*exp(j*Vac_Init(2)*pi/180);
      | u2=Vdc_Init*exp(j*90*pi/180);
      | u=u1+u2;
      | u0=imag(u); % input at  t=0;
      | I=eye(size(Ac));
      | sI1=I*j*(2*pi*Vac_Init(3));
      | sI2=I*j*0;
      | x=inv(sI1-Ac)*Bc*u1 + inv(sI2-Ac)*Bc*u2;
      | x0c=imag(x);
      | x0d=(I-Ac*Ts/2)*x0c/Ts - Bc/2*u0;
      | else
      | x0d=0;
      | end
      | %
      | if PlotResponse==1 % Plot frequency and step response
      | if Zeta==1
      | 	z=1+1e-12;
      | else
      | 	z=Zeta;
      | end
      | wn=Wo;
      | t=[0:1/(z*wn)/1000:7/(z*wn)];
      | f=param1(1):param1(3):param1(2);
      | w=2*pi*f;
      | switch FilterType
      | 	case 1, % Lowpass
      | 		Ystep=wn^2*(1/wn^2+1/(4*z^2*wn^2-4*wn^2)^(1/2)*(1/(-z*wn+1/2*(4*z^2*wn^2-4*wn^2)^(1/2))*exp((-z*wn+1/2*(4*z^2*wn^2-4*wn^2)^(1/2))*t)-1/(-z*wn-1/2*(4*z^2*wn^2-4*wn^2)^(1/2))*exp((-z*wn-1/2*(4*z^2*wn^2-4*wn^2)^(1/2))*t)));
      | 		numFreq=wn^2;
      | 	case 2,   % Highpass
      | 		Ystep=-exp(-z*wn*t)/(z-1)/(z+1).*cos((-wn^2*(z-1)*(z+1))^(1/2)*t)+exp(-z*wn*t)/(z-1)/(z+1)*z^2.*cos((-wn^2*(z-1)*(z+1))^(1/2)*t)+z/wn*exp(-z*wn*t)/(z-1)/(z+1)*(wn^2-z^2*wn^2)^(1/2).*sin((-wn^2*(z-1)*(z+1))^(1/2)*t);
      | 		numFreq=-w.^2;
      | 	case 3,   % Bandpass
      | 		Ystep=2*z*wn/(4*z^2*wn^2-4*wn^2)^(1/2)*(exp((-z*wn+1/2*(4*z^2*wn^2-4*wn^2)^(1/2))*t)-exp((-z*wn-1/2*(4*z^2*wn^2-4*wn^2)^(1/2))*t));
      | 		numFreq=2*Zeta*wn.*w*j;
      | 	case 4,  %Bandstop (Notch)
      | 		Ystep=1+2*z/wn*exp(-z*wn*t)/(z-1)/(z+1)*(wn^2-z^2*wn^2)^(1/2).*sin((-wn^2*(z-1)*(z+1))^(1/2)*t);	
      | 		numFreq=wn^2-w.^2;
      | end
      | %
      | denFreq=(wn^2-w.^2) + 2*Zeta*wn*j.*w;
      | RepFreq=numFreq./denFreq;
      | Mag=abs(RepFreq);
      | Pha=angle(RepFreq)*180/pi;
      | %
      | figure(1)
      | subplot(2,1,1)
      | plot(f,Mag)
      | grid
      | title('Bode Diagram')
      | ylabel('Magnitude')
      | subplot(2,1,2)
      | plot(f,Pha)
      | ylabel('Phase (deg)')
      | xlabel('Frequency (Hz)')
      | grid
      | figure(2)
      | plot(t,real(Ystep))
      | grid
      | ylabel('Amplitude')
      | xlabel('Time (s)')
      | title('Step Response')
      | end
      mask Help: This block is part of a subset of blocks in the Extras library that does not have documentation associated with it, other than the block mask description.
      mask TypeOptions FilterType: Lowpass | Highpass | Bandpass | Bandstop (Notch)
      mask Callback Initialize: p5=get_param(gcb,'Initialize');if strcmp(p5,'on');visible={'on','on','on','on','on','on','on','on',get_param(gcb,'PlotResponse')};else;visible={'on','on','on','on','on','off','off','on',get_param(gcb,'PlotResponse')};end;set_param(gcb,'MaskVisibilities',visible)
      mask Callback PlotResponse: p8=get_param(gcb,'PlotResponse');if strcmp(p8,'on');visible={'on','on','on','on','on',get_param(gcb,'Initialize'),get_param(gcb,'Initialize'),'on','on'};else;visible={'on','on','on','on','on',get_param(gcb,'Initialize'),get_param(gcb,'Initialize'),'on','off'};end;set_param(gcb,'MaskVisibilities',visible)
      mask Display:
      | plot(X,Y);
      | disp(str);
  Automatic Gain Control : Subsystem  TreatAsAtomicUnit=on
  Constant1 : Constant  Value=AGC
  Constant4 : Constant  Value=2*pi
  Controller : Subsystem  mask(Discrete PID Controller){Kp=Kp, Ki=Ki, Kd=Kd, Par_Limits=[10000 0], Init=2*pi*Finit, Ts=Ts}
      mask prompts: Kp "Proportional gain (Kp):"; Ki "Integral gain (Ki):"; Kd "Derivative gain (Kd):"; Par_Limits "Output limits: [ Upper   Lower ]"; Init "Output initial value:"; Ts "Sample time:"
      mask help: This block implements a discrete PID controller.
      mask init:
      | UpperLimit=Par_Limits(1);
      | LowerLimit=Par_Limits(2);
      settings: OpenFcn=power_openblockproxy();
      mask Display: disp('PID');
  Discrete Rate Limiter : Subsystem  mask(Discrete Rate Limiter){R=12, F=-12, Vinit=Finit, Ts=Ts}
      mask prompts: R "Rising slew rate:"; F "Falling slew rate:"; Vinit "Initial input:"; Ts "Sample time:"
      mask init:
      | UpperLimit=R*Ts;
      | LowerLimit=F*Ts;
      mask Display: disp('Discrete\nRate\nLimiter')
  Discrete-Time Integrator : DiscreteIntegrator  InitialCondition=Phase_Init*pi/180  SampleTime=Ts  ICPrevOutput=DiscIntNeverNeededParam  ICPrevScaledInput=DiscIntNeverNeededParam
  Divide : Product
  Gain10 : Gain  Gain=1/2/pi  SaturateOnIntegerOverflow=on  OutDataTypeStr=Inherit: Same as input  ParamDataTypeStr=Inherit: Same as input
  Math Function : Math  Operator=mod  SignedPower=on
  Mux2 : Mux  Inputs=2
  Selector : Selector  InputPortWidth=3  IndexOptions=Index vector (dialog)  Indices=2  OutputSizes=1
  Trigonometric Function : Trigonometry
  Trigonometric Function2 : Trigonometry  Operator=cos
  Unit Delay : UnitDelay  InitialCondition=Finit  SampleTime=Ts  HasFrameUpgradeWarning=on
  Variable Frequency Mean value : Subsystem  mask(Discrete Variable-Frequency Mean Value){Finit=Finit, Fmin=Fmin, Vinit=0, Ts=Ts}
      mask prompts: Finit "Initial frequency (Hz):"; Fmin "Minimum frequency (Hz):"; Vinit "Initial input (DC component):"; Ts "Sample time:"
      mask help: Compute the mean value of input 2 over a running window of one cycle of frequency given by input 1.
      mask init:
      | MaxDelay=1/Fmin+Ts;
      mask Display: disp('')
  abc_to_dq0 Transformation : Subsystem  mask(abc to dq0 Transformation){}
      mask help: Perform a Park transformation from the three-phase (abc) reference frame to the dq0 reference frame.
      mask Display: disp('')
  Freq : Outport  VectorParamsAs1DForOutWhenUnconnected=off
  wt : Outport  Port=2  VectorParamsAs1DForOutWhenUnconnected=off
  Sin_Cos : Outport  Port=3  VectorParamsAs1DForOutWhenUnconnected=off
  wires:
  Selector/1 -> Variable Frequency Mean value/2(In)  "Vq"
  2nd-Order Filter/1(Out) -> Unit Delay/1
  Unit Delay/1 -> Freq/1, Variable Frequency Mean value/1(Freq), Automatic Gain Control/1(Freq)
  Discrete Rate Limiter/1(Out) -> 2nd-Order Filter/1(In)
  Gain10/1 -> Discrete Rate Limiter/1(In)
  Mux2/1 -> Sin_Cos/1, abc_to_dq0 Transformation/2(sin_cos), Automatic Gain Control/2(Sin_Cos)
  Trigonometric Function2/1 -> Mux2/2
  Trigonometric Function/1 -> Mux2/1
  Math Function/1 -> wt/1, Trigonometric Function2/1, Trigonometric Function/1
  Discrete-Time Integrator/1 -> Math Function/1
  Constant4/1 -> Math Function/2
  abc_to_dq0 Transformation/1(dq0) -> Selector/1
  Vabc(pu)/1 -> abc_to_dq0 Transformation/1(abc), Automatic Gain Control/3(Vabc)
  Controller/1(Out) -> Discrete-Time Integrator/1, Gain10/1  "W"
  Variable Frequency Mean value/1(Mean) -> Divide/1
  Automatic Gain Control/1(Gain) -> Divide/2
  Divide/1 -> Controller/1(Error)
  Constant1/1 -> Automatic Gain Control/Enable

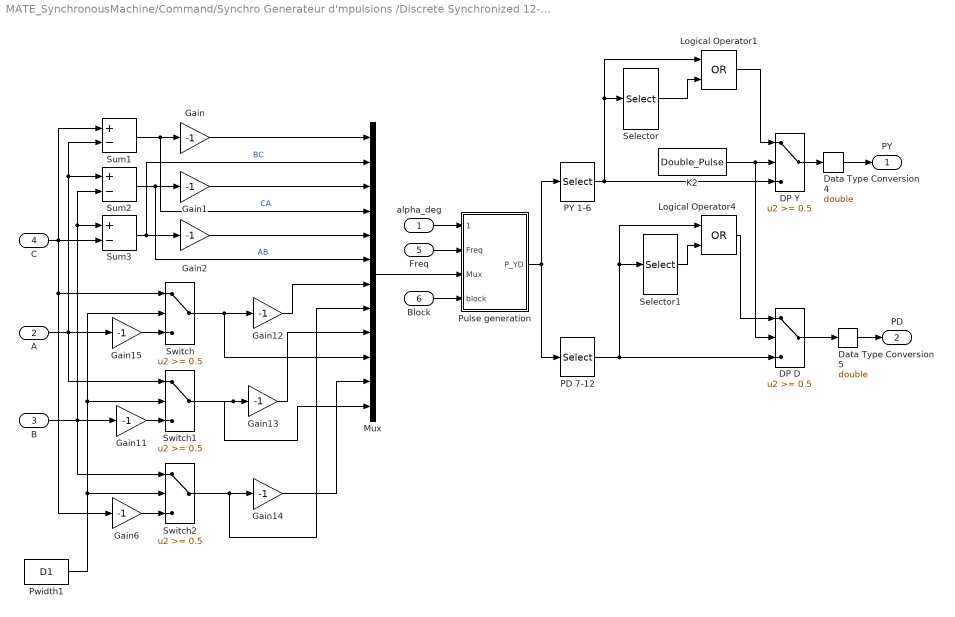
== system MATE_SynchronousMachine/Command/Synchro Generateur d'mpulsions /Discrete Synchronized 12-Pulse Generator ==
  alpha_deg : Inport
  A : Inport  Port=2
  B : Inport  Port=3
  C : Inport  Port=4
  Freq : Inport  Port=5
  Block : Inport  Port=6
  DP D : Switch  Threshold=0.5  SaturateOnIntegerOverflow=off
  DP Y : Switch  Threshold=0.5  SaturateOnIntegerOverflow=off
  Data Type Conversion4 : DataTypeConversion  OutDataTypeStr=double
  Data Type Conversion5 : DataTypeConversion  OutDataTypeStr=double
  Gain{,1..2,6,11..15} (9 alike) : Gain  Gain=-1  SaturateOnIntegerOverflow=on  OutDataTypeStr=Inherit: Same as input  ParamDataTypeStr=Inherit: Same as input
  K2 : Constant  Value=Double_Pulse
  Logical Operator1 : Logic  Operator=OR
  Logical Operator4 : Logic  Operator=OR
  Mux : Mux  Inputs=12
  PD 7-12 : Selector  InputPortWidth=12  IndexOptions=Index vector (dialog)  Indices=7:12  OutputSizes=1
  PY 1-6 : Selector  InputPortWidth=12  IndexOptions=Index vector (dialog)  Indices=1:6  OutputSizes=1
  Pulse generation : Subsystem
  Pwidth1 : Constant  Value=D1
  Selector : Selector  InputPortWidth=6  IndexOptions=Index vector (dialog)  Indices=[2 3 4 5 6 1 ]  OutputSizes=1
  Selector1 : Selector  InputPortWidth=6  IndexOptions=Index vector (dialog)  Indices=[2 3 4 5 6 1 ]  OutputSizes=1
  Sum1 : Sum  Inputs=+-  InputSameDT=on  SaturateOnIntegerOverflow=on  OutDataTypeStr=Inherit: Same as first input
  Sum2 : Sum  Inputs=+-  InputSameDT=on  SaturateOnIntegerOverflow=on  OutDataTypeStr=Inherit: Same as first input
  Sum3 : Sum  Inputs=+-  InputSameDT=on  SaturateOnIntegerOverflow=on  OutDataTypeStr=Inherit: Same as first input
  Switch : Switch  Threshold=0.5  SaturateOnIntegerOverflow=off  InputSameDT=off
  Switch1 : Switch  Threshold=0.5  SaturateOnIntegerOverflow=off  InputSameDT=off
  Switch2 : Switch  Threshold=0.5  SaturateOnIntegerOverflow=off  InputSameDT=off
  PY : Outport  InitialOutput=0  VectorParamsAs1DForOutWhenUnconnected=off
  PD : Outport  Port=2  InitialOutput=0  VectorParamsAs1DForOutWhenUnconnected=off
  wires:
  Pulse generation/1(P_YD) -> PY 1-6/1, PD 7-12/1
  Freq/1 -> Pulse generation/2(Freq)
  alpha_deg/1 -> Pulse generation/1(alpha_deg)
  Logical Operator1/1 -> DP Y/1
  Selector/1 -> Logical Operator1/2
  PY 1-6/1 -> DP Y/3, Selector/1, Logical Operator1/1
  Logical Operator4/1 -> DP D/1
  Selector1/1 -> Logical Operator4/2
  PD 7-12/1 -> Logical Operator4/1, Selector1/1, DP D/3
  K2/1 -> DP Y/2, DP D/2
  Block/1 -> Pulse generation/4(block)
  DP Y/1 -> Data Type Conversion4/1
  Data Type Conversion4/1 -> PY/1
  DP D/1 -> Data Type Conversion5/1
  Data Type Conversion5/1 -> PD/1
  Pwidth1/1 -> Switch2/2, Switch1/2, Switch/2
  Gain14/1 -> Mux/11
  Gain13/1 -> Mux/9
  Gain12/1 -> Mux/7
  Gain6/1 -> Switch2/3
  Gain11/1 -> Switch1/3
  Gain15/1 -> Switch/3
  Switch/1 -> Mux/10, Gain12/1
  Switch2/1 -> Mux/8, Gain14/1
  Switch1/1 -> Mux/12, Gain13/1
  Mux/1 -> Pulse generation/3(Mux)
  Gain2/1 -> Mux/5
  Gain1/1 -> Mux/3
  Gain/1 -> Mux/1
  Sum1/1 -> Gain/1, Mux/4  "CA"
  Sum2/1 -> Gain1/1, Mux/6  "AB"
  Sum3/1 -> Gain2/1, Mux/2  "BC"
  C/1 -> Switch/1, Gain6/1, Sum1/1, Sum3/2
  A/1 -> Switch1/1, Gain15/1, Sum2/1, Sum1/2
  B/1 -> Switch2/1, Sum2/2, Sum3/1, Gain11/1

== system MATE_SynchronousMachine/MATE Synchronous Machine (p=20)/Delta angle/Cartesian to Polar ==
  x : Inport
  y : Inport  Port=2
  Mux : Mux  Inputs=2
  x->r : Fcn  Expr=hypot(u[1],u[2])
  x->theta : Fcn  Expr=atan2(u[2],u[1])
  r : Outport  InitialOutput=0
  theta : Outport  Port=2  InitialOutput=0
  wires:
  Mux/1 -> x->theta/1, x->r/1
  x->r/1 -> r/1
  x/1 -> Mux/1
  y/1 -> Mux/2
  x->theta/1 -> theta/1

== system MATE_SynchronousMachine/MATE Synchronous Machine (p=20)/Delta angle/Radians to Degrees ==
  Radians in : Inport
  Gain : Gain  Gain=180/pi  SaturateOnIntegerOverflow=on  OutDataTypeStr=Inherit: Same as input  ParamDataTypeStr=Inherit: Same as input
  Degrees out : Outport  InitialOutput=0
  wires:
  Gain/1 -> Degrees out/1
  Radians in/1 -> Gain/1

== system MATE_SynchronousMachine/MATE Synchronous Machine (p=20)/SSS-SM equations/Discretize ==
  Ac : Inport
  Bc : Inport  Port=2
  Unity : Inport  Port=3
  Product1 : Product  Multiplication=Matrix(*)  SaturateOnIntegerOverflow=on  OutDataTypeStr=Inherit: Same as first input
  Product2 : Product  Multiplication=Matrix(*)  SaturateOnIntegerOverflow=on  OutDataTypeStr=Inherit: Same as first input
  Product4 : Product  Multiplication=Matrix(*)  SaturateOnIntegerOverflow=on  OutDataTypeStr=Inherit: Same as first input
  Sum1 : Sum  Inputs=+-  SaturateOnIntegerOverflow=on
  Sum5 : Sum  SaturateOnIntegerOverflow=on
  Ts/2 : Gain  Gain=Ts/2  SaturateOnIntegerOverflow=on  OutDataTypeStr=Inherit: Same as input  ParamDataTypeStr=Inherit: Same as input
  inversion : Product  Inputs=/  Multiplication=Matrix(*)  RndMeth=Zero
  trapeze has Ts/2 factor on B : Gain  Gain=Ts/2  SaturateOnIntegerOverflow=on  OutDataTypeStr=Inherit: Same as input  ParamDataTypeStr=Inherit: Same as input
  trapeze has Ts/2 factor on B1 : Gain  Gain=Ts/2  SaturateOnIntegerOverflow=on  OutDataTypeStr=Inherit: Same as input  ParamDataTypeStr=Inherit: Same as input
  Ad : Outport
  Bd : Outport  Port=2
  Bdin : Outport  Port=3
  wires:
  Sum1/1 -> inversion/1
  Ac/1 -> Ts/2/1
  Product1/1 -> Bd/1
  Sum5/1 -> Product4/2
  Unity/1 -> Sum1/1, Sum5/1, trapeze has Ts/2 factor on B1/1
  Product4/1 -> Ad/1
  Ts/2/1 -> Sum1/2, Sum5/2
  trapeze has Ts/2 factor on B/1 -> Product1/2
  Bc/1 -> trapeze has Ts/2 factor on B/1
  inversion/1 -> Product4/1, Product1/1, Product2/1  "inv(I4-Ts/2*A)"
  Product2/1 -> Bdin/1
  trapeze has Ts/2 factor on B1/1 -> Product2/2

== system MATE_SynchronousMachine/MATE Synchronous Machine (p=20)/SSS-SM equations/Subsystem1 ==
  In1 : Inport
  Demux : Demux  Outputs=[5 1 ]
  Mux : Mux  Inputs=2
  u1 : Constant  Value=0
  Out1 : Outport
  wires:
  In1/1 -> Demux/1
  u1/1 -> Mux/2
  Demux/1 -> Mux/1
  Mux/1 -> Out1/1

== system MATE_SynchronousMachine/MATE Synchronous Machine (p=20)/SSS-SM equations zero sequence only/Discretize ==
  Ac : Inport
  Bc : Inport  Port=2
  Unity : Inport  Port=3
  Product1 : Product  Multiplication=Matrix(*)  SaturateOnIntegerOverflow=on  OutDataTypeStr=Inherit: Same as first input
  Product4 : Product  Multiplication=Matrix(*)  SaturateOnIntegerOverflow=on  OutDataTypeStr=Inherit: Same as first input
  Sum1 : Sum  Inputs=+-  SaturateOnIntegerOverflow=on
  Sum5 : Sum  SaturateOnIntegerOverflow=on
  Ts/2 : Gain  Gain=Ts/2  SaturateOnIntegerOverflow=on  OutDataTypeStr=Inherit: Same as input  ParamDataTypeStr=Inherit: Same as input
  inversion : Product  Inputs=/  Multiplication=Matrix(*)  RndMeth=Zero
  trapeze has Ts/2 factor on B : Gain  Gain=Ts/2  SaturateOnIntegerOverflow=on  OutDataTypeStr=Inherit: Same as input  ParamDataTypeStr=Inherit: Same as input
  Ad : Outport
  Bd : Outport  Port=2
  wires:
  Sum1/1 -> inversion/1
  Ac/1 -> Ts/2/1
  Product1/1 -> Bd/1
  Sum5/1 -> Product4/2
  Unity/1 -> Sum1/1, Sum5/1
  Product4/1 -> Ad/1
  Ts/2/1 -> Sum1/2, Sum5/2
  trapeze has Ts/2 factor on B/1 -> Product1/2
  Bc/1 -> trapeze has Ts/2 factor on B/1
  inversion/1 -> Product1/1, Product4/1  "inv(I4-Ts/2*A)"

== system MATE_SynchronousMachine/MATE Synchronous Machine (p=20)/Saturation/Lad ==
  note: Lad =1/(1/Lmd+1/Ll+1/Llkd+1/Llfd)
  Lmd : Inport
  Math Function2 : Math  Operator=reciprocal  SignedPower=on
  Math Function3 : Math  Operator=reciprocal  SignedPower=on
  Mux2 : Mux  Inputs=[3 1]
  Sum1 : Sum  Inputs=+  SaturateOnIntegerOverflow=on
  u1 : Constant  Value=[1/Lls 1/Llkd 1/Llf]
  Lad : Outport
  wires:
  u1/1 -> Mux2/1
  Mux2/1 -> Sum1/1
  Sum1/1 -> Math Function3/1
  Math Function3/1 -> Lad/1
  Lmd/1 -> Math Function2/1
  Math Function2/1 -> Mux2/2

== system MATE_SynchronousMachine/MATE Synchronous Machine (p=20)/Saturation/Laq ==
  note: Laq = 1/(1/Lmq+1Ll+1/Llkq1+1/Llkq2)
  Lmq : Inport
  Math Function : Math  Operator=reciprocal  SignedPower=on
  Math Function1 : Math  Operator=reciprocal  SignedPower=on
  Mux1 : Mux  Inputs=[3 1]
  Sum2 : Sum  Inputs=+  SaturateOnIntegerOverflow=on
  u2 : Constant  Value=[ 1/Lls 1/Llkq 1/Llkq2]
  Laq : Outport
  wires:
  Math Function/1 -> Mux1/2
  Lmq/1 -> Math Function/1
  Math Function1/1 -> Laq/1
  Sum2/1 -> Math Function1/1
  Mux1/1 -> Sum2/1
  u2/1 -> Mux1/1

== system MATE_SynchronousMachine/MATE Synchronous Machine (p=20)/Saturation/phimd ==
  note: phimd= phids*(Lad/Lls) +phifd*(Lad/Llfd) + phikd*(Lad/Llkd)
  phi : Inport
  Lad : Inport  Port=2
  1/Ll_d : Gain  Gain="[ 1/Lls   1/Llf   1/Llkd ]"  SaturateOnIntegerOverflow=on  OutDataTypeStr=Inherit: Same as input  ParamDataTypeStr=Inherit: Same as input
  Product4 : Product  RndMeth=Zero
  "phid phifd phikd " : Selector  InputPortWidth=7  IndexOptions=Index vector (dialog)  Indices=[1 3 4]  OutputSizes=1
  sum2 : Sum  Inputs=+  InputSameDT=on  SaturateOnIntegerOverflow=on  OutDataTypeStr=Inherit: Same as first input
  phimd : Outport
  wires:
  sum2/1 -> Product4/1  "phimd"
  "phid phifd phikd "/1 -> 1/Ll_d/1
  1/Ll_d/1 -> sum2/1
  phi/1 -> "phid phifd phikd "/1
  Product4/1 -> phimd/1  "phimd"
  Lad/1 -> Product4/2

== system MATE_SynchronousMachine/MATE Synchronous Machine (p=20)/Saturation/phimq ==
  note: phimq= phiqs*(Laq/Lls) +phikq1*(Laq/Llkq1) +phikq2*(Laq/Llkq2)
  Laq : Inport
  phi : Inport  Port=2
  1/Ll_q : Gain  Gain=[1/Lls 1/Llkq 1/Llkq2]  SaturateOnIntegerOverflow=on  OutDataTypeStr=Inherit: Same as input  ParamDataTypeStr=Inherit: Same as input
  Product3 : Product  RndMeth=Zero
  phiq phikq1 (phikq2) : Selector  InputPortWidth=7  IndexOptions=Index vector (dialog)  Indices=[2 5 6]  OutputSizes=1
  sum1 : Sum  Inputs=+  InputSameDT=on  SaturateOnIntegerOverflow=on  OutDataTypeStr=Inherit: Same as first input
  phimq : Outport
  wires:
  1/Ll_q/1 -> sum1/1
  phiq phikq1 (phikq2)/1 -> 1/Ll_q/1
  sum1/1 -> Product3/1  "phimq"
  Laq/1 -> Product3/2
  Product3/1 -> phimq/1  "phimq"
  phi/1 -> phiq phikq1 (phikq2)/1

== system MATE_SynchronousMachine/MATE_LineCommutatedConverter/MATEPREP/RCsnuber ==
  Capacitor : fl_lib/Electrical/Electrical Elements/Capacitor  c=Csnu F  r=0 Ohm  g=0 1/Ohm  i_specify=off  i_priority=None  i=0 A  i_nominal_specify=off  i_nominal_value=1  i_nominal_unit=A  v_specify=off  v_priority=None  v=0 V  v_nominal_specify=off  v_nominal_value=1  v_nominal_unit=V  vc_specify=off  vc_priority=High  vc=0 V  vc_nominal_specify=off  vc_nominal_value=1  vc_nominal_unit=V
  Resistor : fl_lib/Electrical/Electrical Elements/Resistor  R=Rsnu Ohm  i_specify=off  i_priority=None  i=0 A  i_nominal_specify=off  i_nominal_value=1  i_nominal_unit=A  v_specify=off  v_priority=None  v=0 V  v_nominal_specify=off  v_nominal_value=1  v_nominal_unit=V
  + : PMIOPort  Side=Left
  - : PMIOPort  Port=2  Side=Right
  connections:
  Resistor/LConn1 -- Capacitor/RConn1
  Capacitor/LConn1 -- +/RConn1
  Resistor/RConn1 -- -/RConn1

== system MATE_SynchronousMachine/MATE_LineCommutatedConverter/MATEPREP/RCsnuber1 ==
  Capacitor : fl_lib/Electrical/Electrical Elements/Capacitor  c=Csnu F  r=0 Ohm  g=0 1/Ohm  i_specify=off  i_priority=None  i=0 A  i_nominal_specify=off  i_nominal_value=1  i_nominal_unit=A  v_specify=off  v_priority=None  v=0 V  v_nominal_specify=off  v_nominal_value=1  v_nominal_unit=V  vc_specify=off  vc_priority=High  vc=0 V  vc_nominal_specify=off  vc_nominal_value=1  vc_nominal_unit=V
  Resistor : fl_lib/Electrical/Electrical Elements/Resistor  R=Rsnu Ohm  i_specify=off  i_priority=None  i=0 A  i_nominal_specify=off  i_nominal_value=1  i_nominal_unit=A  v_specify=off  v_priority=None  v=0 V  v_nominal_specify=off  v_nominal_value=1  v_nominal_unit=V
  + : PMIOPort  Side=Left
  - : PMIOPort  Port=2  Side=Right
  connections:
  Resistor/RConn1 -- -/RConn1
  Capacitor/LConn1 -- +/RConn1
  Resistor/LConn1 -- Capacitor/RConn1

== system MATE_SynchronousMachine/MATE_LineCommutatedConverter/MATEPREP/RCsnuber2 ==
  Capacitor : fl_lib/Electrical/Electrical Elements/Capacitor  c=Csnu F  r=0 Ohm  g=0 1/Ohm  i_specify=off  i_priority=None  i=0 A  i_nominal_specify=off  i_nominal_value=1  i_nominal_unit=A  v_specify=off  v_priority=None  v=0 V  v_nominal_specify=off  v_nominal_value=1  v_nominal_unit=V  vc_specify=off  vc_priority=High  vc=0 V  vc_nominal_specify=off  vc_nominal_value=1  vc_nominal_unit=V
  Resistor : fl_lib/Electrical/Electrical Elements/Resistor  R=Rsnu Ohm  i_specify=off  i_priority=None  i=0 A  i_nominal_specify=off  i_nominal_value=1  i_nominal_unit=A  v_specify=off  v_priority=None  v=0 V  v_nominal_specify=off  v_nominal_value=1  v_nominal_unit=V
  + : PMIOPort  Side=Left
  - : PMIOPort  Port=2  Side=Right
  connections:
  Resistor/LConn1 -- Capacitor/RConn1
  Capacitor/LConn1 -- +/RConn1
  Resistor/RConn1 -- -/RConn1

== system MATE_SynchronousMachine/MATE_LineCommutatedConverter/MATEPREP/RCsnuber3 ==
  Capacitor : fl_lib/Electrical/Electrical Elements/Capacitor  c=Csnu F  r=0 Ohm  g=0 1/Ohm  i_specify=off  i_priority=None  i=0 A  i_nominal_specify=off  i_nominal_value=1  i_nominal_unit=A  v_specify=off  v_priority=None  v=0 V  v_nominal_specify=off  v_nominal_value=1  v_nominal_unit=V  vc_specify=off  vc_priority=High  vc=0 V  vc_nominal_specify=off  vc_nominal_value=1  vc_nominal_unit=V
  Resistor : fl_lib/Electrical/Electrical Elements/Resistor  R=Rsnu Ohm  i_specify=off  i_priority=None  i=0 A  i_nominal_specify=off  i_nominal_value=1  i_nominal_unit=A  v_specify=off  v_priority=None  v=0 V  v_nominal_specify=off  v_nominal_value=1  v_nominal_unit=V
  + : PMIOPort  Side=Left
  - : PMIOPort  Port=2  Side=Right
  connections:
  Resistor/RConn1 -- -/RConn1
  Capacitor/LConn1 -- +/RConn1
  Resistor/LConn1 -- Capacitor/RConn1
